simulink model "RBCM_Model"  (R2024b)
settings: Solver=FixedStepAuto  StartTime=0.0  StopTime=10.0  RelTol=1e-3
PreLoadFcn:
  | % NXP_MBDT_S32K3 callback: DO NOT REMOVE
  | mbd_s32k3.common.nxp.model_callbacks.preLoadFcn();
PostLoadFcn:
  | % NXP_MBDT_S32K3 callback: DO NOT REMOVE
  | mbd_s32k3.common.nxp.model_callbacks.postLoadFcn();
InitFcn:
  | % NXP_MBDT_S32K3 callback: DO NOT REMOVE
  | mbd_s32k3.common.nxp.model_callbacks.initFcn();
undefined symbols (not defined in the file or in its folder): AccuFanPwr_hHsd3ch2, BspdPwr_lHsd1ch2, BuzzerPwr_lHsd3ch3, DevicePwr_12v_lHsd1ch1, DevicePwr_hHsd1ch2, DrsPwr_8v_lHsd3ch1, hHsd_Diagnose_AdcBuffer, ILPwr_hHsd1ch1, lHsd_Diagnose_AdcBuffer, LoggerPwr_lHsd1ch3, PumpFan1_hHsd4ch1, PumpFan2_hHsd4ch2, PumpPwr_hHsd3ch1, RGBLED0state, TaillightPwr_lHsd3ch4, TempSensorPwr_lHsd1ch4
libraries: mbd_s32k3_io_library x127, simulink x48, canmsglib x8, mbd_s32k3_communication_library x7, mbd_s32k3_isr_library x6, mbd_s32k3_cdd_library x3, mbd_s32k3_utility_library x1
(part 10 of 10)

== matlab function RBCM_Model/HSD诊断分析子系统/错误码转存单元2 ==
  data: index input uint8; u input uint8; y1 output uint8; y2 output uint8; y3 output uint8; y4 output uint8
function [y1, y2, y3, y4] = fcn2(index, u)

% 函数内部声明 可持续类型变量
persistent Y1 Y2 Y3 Y4
% 首先要判断persistent声明的变量是否是空
if isempty(Y1)
    Y1=uint8(0);
    Y2=uint8(0);
    Y3=uint8(0);
    Y4=uint8(0);
end

if index==0
    y1=u;
    y2=Y2;
    y3=Y3;
    y4=Y4;
elseif index==1
    y1=Y1;
    y2=u;
    y3=Y3;
    y4=Y4;
elseif index==2
    y1=Y1;
    y2=Y2;
    y3=u;
    y4=Y4;
elseif index==3
    y1=Y1;
    y2=Y2;
    y3=Y3;
    y4=u;
else
    y1=Y1;
    y2=Y2;
    y3=Y3;
    y4=Y4;
end

Y1=y1;
Y2=y2;
Y3=y3;
Y4=y4;

end

== stateflow chart RBCM_Model/控制状态机/Chart1 ==
  state A
  state A1
  (default) -> A
  A -> A1
  A1 -> A
  data: A output boolean [0..1]

== matlab function RBCM_Model/HSD诊断分析子系统/错误码转存单元3 ==
  data: index input uint8; u input uint8; y1 output uint8; y2 output uint8; y3 output uint8; y4 output uint8
function [y1, y2, y3, y4] = fcn2(index, u)

% 函数内部声明 可持续类型变量
persistent Y1 Y2 Y3 Y4
% 首先要判断persistent声明的变量是否是空
if isempty(Y1)
    Y1=uint8(0);
    Y2=uint8(0);
    Y3=uint8(0);
    Y4=uint8(0);
end

if index==0
    y1=u;
    y2=Y2;
    y3=Y3;
    y4=Y4;
elseif index==1
    y1=Y1;
    y2=u;
    y3=Y3;
    y4=Y4;
elseif index==2
    y1=Y1;
    y2=Y2;
    y3=u;
    y4=Y4;
elseif index==3
    y1=Y1;
    y2=Y2;
    y3=Y3;
    y4=u;
else
    y1=Y1;
    y2=Y2;
    y3=Y3;
    y4=Y4;
end

Y1=y1;
Y2=y2;
Y3=y3;
Y4=y4;

end

== matlab function RBCM_Model/HSD诊断分析子系统/触发器5 ==
  data: y output uint8; counter input uint8; u2 input uint8
  events: fcncall output FUNCTION_CALL_EVENT
function y = fcn(counter,u2)

% 函数内部声明 可持续类型变量 output
persistent i
persistent output  
% 首先要判断persistent声明的变量是否是空
if isempty(i)
    i  = 0;
end
if isempty(output)
    output  = 0;
end

% 自递增
i=i+1;
output=output+1;

%分频计数值溢出
if i>=counter
    %输出值溢出
    if output>=u2
        output=0;
    end

    %输出值
    y = uint8(output);

    %生成触发，触发ADC采集
    fcncall;

    i=0;
else
    y=uint8(output);    %不生成触发
end

end

== matlab function RBCM_Model/HSD诊断分析子系统/诊断数据转存单元5 ==
  data: index input uint8; u input uint16; y1 output uint16; y2 output uint16; y3 output uint16; y4 output uint16
function [y1, y2, y3, y4] = fcn2(index, u)

% 函数内部声明 可持续类型变量
persistent Y1 Y2 Y3 Y4
% 首先要判断persistent声明的变量是否是空
if isempty(Y1)
    Y1=uint16(0);
    Y2=uint16(0);
    Y3=uint16(0);
    Y4=uint16(0);
end

if index==0
    y1=u;
    y2=Y2;
    y3=Y3;
    y4=Y4;
elseif index==1
    y1=Y1;
    y2=u;
    y3=Y3;
    y4=Y4;
elseif index==2
    y1=Y1;
    y2=Y2;
    y3=u;
    y4=Y4;
elseif index==3
    y1=Y1;
    y2=Y2;
    y3=Y3;
    y4=u;
else
    y1=Y1;
    y2=Y2;
    y3=Y3;
    y4=Y4;
end

Y1=y1;
Y2=y2;
Y3=y3;
Y4=y4;

end

== matlab function RBCM_Model/HSD诊断分析子系统/错误码转存单元4 ==
  data: index input uint8; u input uint8; y1 output uint8; y2 output uint8; y3 output uint8; y4 output uint8
function [y1, y2, y3, y4] = fcn2(index, u)

% 函数内部声明 可持续类型变量
persistent Y1 Y2 Y3 Y4
% 首先要判断persistent声明的变量是否是空
if isempty(Y1)
    Y1=uint8(0);
    Y2=uint8(0);
    Y3=uint8(0);
    Y4=uint8(0);
end

if index==0
    y1=u;
    y2=Y2;
    y3=Y3;
    y4=Y4;
elseif index==1
    y1=Y1;
    y2=u;
    y3=Y3;
    y4=Y4;
elseif index==2
    y1=Y1;
    y2=Y2;
    y3=u;
    y4=Y4;
elseif index==3
    y1=Y1;
    y2=Y2;
    y3=Y3;
    y4=u;
else
    y1=Y1;
    y2=Y2;
    y3=Y3;
    y4=Y4;
end

Y1=y1;
Y2=y2;
Y3=y3;
Y4=y4;

end

== matlab function RBCM_Model/HSD诊断分析子系统/数据转存单元2 ==
  data: index input uint8; u input uint8; y1 output uint8; y2 output uint8
function [y1, y2] = fcn2(index, u)

% 函数内部声明 可持续类型变量
persistent Y1 Y2
% 首先要判断persistent声明的变量是否是空
if isempty(Y1)
    Y1=uint8(0);
    Y2=uint8(0);
end

if index==0
    y1=u;
    y2=Y2;
elseif index==1
    y1=Y1;
    y2=u;
else
    y1=Y1;
    y2=Y2;
end

Y1=y1;
Y2=y2;

end

== matlab function RBCM_Model/HSD诊断分析子系统/数据转存单元3 ==
  data: index input uint8; u input uint16; y1 output uint16; y2 output uint16
function [y1, y2] = fcn2(index, u)

% 函数内部声明 可持续类型变量
persistent Y1 Y2
% 首先要判断persistent声明的变量是否是空
if isempty(Y1)
    Y1=uint16(0);
    Y2=uint16(0);
end

if index==0
    y1=u;
    y2=Y2;
elseif index==1
    y1=Y1;
    y2=u;
else
    y1=Y1;
    y2=Y2;
end

Y1=y1;
Y2=y2;

end

== matlab function RBCM_Model/HSD诊断分析子系统/触发器6 ==
  data: y output uint8; counter input uint8; u2 input uint8
  events: fcncall output FUNCTION_CALL_EVENT
function y = fcn(counter,u2)

% 函数内部声明 可持续类型变量 output
persistent i
persistent output  
% 首先要判断persistent声明的变量是否是空
if isempty(i)
    i  = 0;
end
if isempty(output)
    output  = 0;
end

% 自递增
i=i+1;
output=output+1;

%分频计数值溢出
if i>=counter
    %输出值溢出
    if output>=u2
        output=0;
    end

    %输出值
    y = uint8(output);

    %生成触发，触发ADC采集
    fcncall;

    i=0;
else
    y=uint8(output);    %不生成触发
end

end

== matlab function RBCM_Model/HSD诊断分析子系统/数据转存单元4 ==
  data: index input uint8; u input uint8; y1 output uint8; y2 output uint8
function [y1, y2] = fcn2(index, u)

% 函数内部声明 可持续类型变量
persistent Y1 Y2
% 首先要判断persistent声明的变量是否是空
if isempty(Y1)
    Y1=uint8(0);
    Y2=uint8(0);
end

if index==0
    y1=u;
    y2=Y2;
elseif index==1
    y1=Y1;
    y2=u;
else
    y1=Y1;
    y2=Y2;
end

Y1=y1;
Y2=y2;

end

== stateflow chart RBCM_Model/指令报文解码器/Chart1 ==
  state A
  state A1
  (default) -> A
  A -> A1
  A1 -> A
  data: A output boolean [0..1]

== matlab function RBCM_Model/HSD诊断分析子系统/数据转存单元5 ==
  data: index input uint8; u input uint16; y1 output uint16; y2 output uint16
function [y1, y2] = fcn2(index, u)

% 函数内部声明 可持续类型变量
persistent Y1 Y2
% 首先要判断persistent声明的变量是否是空
if isempty(Y1)
    Y1=uint16(0);
    Y2=uint16(0);
end

if index==0
    y1=u;
    y2=Y2;
elseif index==1
    y1=Y1;
    y2=u;
else
    y1=Y1;
    y2=Y2;
end

Y1=y1;
Y2=y2;

end

== matlab function RBCM_Model/HSD诊断分析子系统/数据转存单元6 ==
  data: index input uint8; u input uint8; y1 output uint8; y2 output uint8
function [y1, y2] = fcn2(index, u)

% 函数内部声明 可持续类型变量
persistent Y1 Y2
% 首先要判断persistent声明的变量是否是空
if isempty(Y1)
    Y1=uint8(0);
    Y2=uint8(0);
end

if index==0
    y1=u;
    y2=Y2;
elseif index==1
    y1=Y1;
    y2=u;
else
    y1=Y1;
    y2=Y2;
end

Y1=y1;
Y2=y2;

end

== matlab function RBCM_Model/HSD诊断分析子系统/数据转存单元7 ==
  data: index input uint8; u input uint16; y1 output uint16; y2 output uint16
function [y1, y2] = fcn2(index, u)

% 函数内部声明 可持续类型变量
persistent Y1 Y2
% 首先要判断persistent声明的变量是否是空
if isempty(Y1)
    Y1=uint16(0);
    Y2=uint16(0);
end

if index==0
    y1=u;
    y2=Y2;
elseif index==1
    y1=Y1;
    y2=u;
else
    y1=Y1;
    y2=Y2;
end

Y1=y1;
Y2=y2;

end

== matlab function RBCM_Model/HSD诊断分析子系统/触发器7 ==
  data: y output uint8; counter input uint8; u2 input uint8
  events: fcncall output FUNCTION_CALL_EVENT
function y = fcn(counter,u2)

% 函数内部声明 可持续类型变量 output
persistent i
persistent output  
% 首先要判断persistent声明的变量是否是空
if isempty(i)
    i  = 0;
end
if isempty(output)
    output  = 0;
end

% 自递增
i=i+1;
output=output+1;

%分频计数值溢出
if i>=counter
    %输出值溢出
    if output>=u2
        output=0;
    end

    %输出值
    y = uint8(output);

    %生成触发，触发ADC采集
    fcncall;

    i=0;
else
    y=uint8(output);    %不生成触发
end

end

== matlab function RBCM_Model/HSD诊断分析子系统/触发器8 ==
  data: y output uint8; counter input uint8; u2 input uint8
  events: fcncall output FUNCTION_CALL_EVENT
function y = fcn(counter,u2)

% 函数内部声明 可持续类型变量 output
persistent i
persistent output  
% 首先要判断persistent声明的变量是否是空
if isempty(i)
    i  = 0;
end
if isempty(output)
    output  = 0;
end

% 自递增
i=i+1;
output=output+1;

%分频计数值溢出
if i>=counter
    %输出值溢出
    if output>=u2
        output=0;
    end

    %输出值
    y = uint8(output);

    %生成触发，触发ADC采集
    fcncall;

    i=0;
else
    y=uint8(output);    %不生成触发
end

end

== matlab function RBCM_Model/HSD诊断分析子系统/数据转存单元8 ==
  data: index input uint8; u input uint8; y1 output uint8; y2 output uint8
function [y1, y2] = fcn2(index, u)

% 函数内部声明 可持续类型变量
persistent Y1 Y2
% 首先要判断persistent声明的变量是否是空
if isempty(Y1)
    Y1=uint8(0);
    Y2=uint8(0);
end

if index==0
    y1=u;
    y2=Y2;
elseif index==1
    y1=Y1;
    y2=u;
else
    y1=Y1;
    y2=Y2;
end

Y1=y1;
Y2=y2;

end

== matlab function RBCM_Model/HSD诊断分析子系统/数据转存单元9 ==
  data: index input uint8; u input uint16; y1 output uint16; y2 output uint16
function [y1, y2] = fcn2(index, u)

% 函数内部声明 可持续类型变量
persistent Y1 Y2
% 首先要判断persistent声明的变量是否是空
if isempty(Y1)
    Y1=uint16(0);
    Y2=uint16(0);
end

if index==0
    y1=u;
    y2=Y2;
elseif index==1
    y1=Y1;
    y2=u;
else
    y1=Y1;
    y2=Y2;
end

Y1=y1;
Y2=y2;

end

== matlab function RBCM_Model/HSD诊断分析子系统/触发器9 ==
  data: y output uint8; counter input uint8; u2 input uint8
  events: fcncall output FUNCTION_CALL_EVENT
function y = fcn(counter,u2)

% 函数内部声明 可持续类型变量 output
persistent i
persistent output  
% 首先要判断persistent声明的变量是否是空
if isempty(i)
    i  = 0;
end
if isempty(output)
    output  = 0;
end

% 自递增
i=i+1;
output=output+1;

%分频计数值溢出
if i>=counter
    %输出值溢出
    if output>=u2
        output=0;
    end

    %输出值
    y = uint8(output);

    %生成触发，触发ADC采集
    fcncall;

    i=0;
else
    y=uint8(output);    %不生成触发
end

end

== matlab function RBCM_Model/HSD诊断分析子系统/数据转存单元10 ==
  data: index input uint8; u input uint8; y1 output uint8; y2 output uint8
function [y1, y2] = fcn2(index, u)

% 函数内部声明 可持续类型变量
persistent Y1 Y2
% 首先要判断persistent声明的变量是否是空
if isempty(Y1)
    Y1=uint8(0);
    Y2=uint8(0);
end

if index==0
    y1=u;
    y2=Y2;
elseif index==1
    y1=Y1;
    y2=u;
else
    y1=Y1;
    y2=Y2;
end

Y1=y1;
Y2=y2;

end

== stateflow chart RBCM_Model/HSD驱动子系统/Subsystem1/Chart19 ==
  settings: description=寄存上一次的操作状态，同则不再操作，异才操作
  state High
    en:register=1
    du:register=1
  state Low
    en:register=0
    du:register=0
  (default) -> High
  High -> Low : [[bit==0]&[bit~=bit0]]{bit0=bit}
  Low -> High : [[bit==1]&[bit~=bit0]]{bit0=bit}
  data: bit input; register output

== matlab function RBCM_Model/HSD诊断分析子系统/数据转存单元12 ==
  data: index input uint8; u input uint16; y1 output uint16; y2 output uint16
function [y1, y2] = fcn2(index, u)

% 函数内部声明 可持续类型变量
persistent Y1 Y2
% 首先要判断persistent声明的变量是否是空
if isempty(Y1)
    Y1=uint16(0);
    Y2=uint16(0);
end

if index==0
    y1=u;
    y2=Y2;
elseif index==1
    y1=Y1;
    y2=u;
else
    y1=Y1;
    y2=Y2;
end

Y1=y1;
Y2=y2;

end

== matlab function RBCM_Model/HSD诊断分析子系统/触发器10 ==
  data: y output uint8; counter input uint8; u2 input uint8
  events: fcncall output FUNCTION_CALL_EVENT
function y = fcn(counter,u2)

% 函数内部声明 可持续类型变量 output
persistent i
persistent output  
% 首先要判断persistent声明的变量是否是空
if isempty(i)
    i  = 0;
end
if isempty(output)
    output  = 0;
end

% 自递增
i=i+1;
output=output+1;

%分频计数值溢出
if i>=counter
    %输出值溢出
    if output>=u2
        output=0;
    end

    %输出值
    y = uint8(output);

    %生成触发，触发ADC采集
    fcncall;

    i=0;
else
    y=uint8(output);    %不生成触发
end

end

== stateflow chart RBCM_Model/4G通信控制状态机1 ==
  settings: executeAtInitialization=1
  state init
    counter=0;
  state first
    if signal==0
    output=A
    counter = counter + 1
    end
  state second
    if signal==0
    output=B
    counter = counter + 1
    end
  state third
    if signal==0
    output=C
    counter = counter + 1
    end
  state fourth
    if signal==0
    output=D
    counter = counter + 1
    end
  state msgsend
  (default) -> init
  init -> first : timer_event[enable==1]{output=A}
  first -> init [order 2] : [enable==0||counter>=5]
  first -> second [order 1] : timer_event[signal==2]{output=B,counter=0}
  msgsend -> init [order 1] : [enable==0||counter>=5]
  fourth -> init [order 2] : [enable==0||counter>=5]
  second -> init [order 1] : [enable==0||counter>=5]
  second -> third [order 2] : timer_event[signal==2]{output=C,counter=0}
  third -> fourth : timer_event[signal==2]{output=D,counter=0}
  fourth -> msgsend [order 1] : timer_event[signal==2]{output=stringin,counter=0}
  msgsend -> msgsend [order 2] : timer_event{output=stringin}
  data: signal input uint32; enable input uint8; B local string ='AT+QMTOPEN=0,"2ac4d9928b.st1.iotda-device.cn-east-3.myhuaweicloud.com",1883'; C local string ='AT+QMTCONN=0,"E10_10101010_0_0_2024112708","E10_10101010","70cb096b1e95f2f5f6fa4a703d88b56f5d4bc5062f406b1091639f697a62929d"'; D local string ='AT+QMTSUB=0,1,"wute/car/test",2'; output output string; stringin input string; counter local uint8 size=1; A local string ="AT"
  events: timer_event input FUNCTION_CALL_EVENT

== matlab function RBCM_Model/Subsystem13/Subsystem/HsdDriveCommand Struct1 ==
  data: HsdDriveCommands output Bus: Bus_Hsd_Drive_Commands
function HsdDriveCommands = fcn

HsdDriveCommands.DevicePwr_12v_lHsd1ch1 = uint8(1);
HsdDriveCommands.BspdPwr_lHsd1ch2 = uint8(1);
HsdDriveCommands.LoggerPwr_lHsd1ch3 = uint8(1);
HsdDriveCommands.TempSensorPwr_lHsd1ch4 = uint8(1);

HsdDriveCommands.DevicePwr_12v_lHsd2ch1 = uint8(1);
HsdDriveCommands.VcuPwr_lHsd2ch2 = uint8(1);
HsdDriveCommands.Fireon_Pwr_lHsd2ch3 = uint8(1);
HsdDriveCommands.DsbdPwr_lHsd2ch4 = uint8(1);

HsdDriveCommands.DrsPwr_8v_lHsd3ch1 = uint8(1);
HsdDriveCommands.DevicePwr_lHsd3ch2 = uint8(1);
HsdDriveCommands.BuzzerPwr_lHsd3ch3 = uint8(1);
HsdDriveCommands.TaillightPwr_lHsd3ch4 = uint8(1);

HsdDriveCommands.DevicePwr_5v_lHsd4ch1 = uint8(1);
HsdDriveCommands.AccuUbr_lHsd4ch2 = uint8(1);
HsdDriveCommands.AccuPwr_lHsd4ch3 = uint8(1);
HsdDriveCommands.BduPwr_lHsd4ch4 = uint8(1);

HsdDriveCommands.DevicePwr_5v_lHsd5ch1 = uint8(1);
HsdDriveCommands.McuUbr_lHsd5ch2 = uint8(1);
HsdDriveCommands.EnergeMeterPwr_lHsd5ch3 = uint8(1);
HsdDriveCommands.TsalrPwr_lHsd5ch4 = uint8(1);


HsdDriveCommands.ILPwr_hHsd1ch1 = uint8(1);
HsdDriveCommands.DevicePwr_hHsd1ch2 = uint8(1);

HsdDriveCommands.VcuUbr_hHsd2ch1 = uint8(1);
HsdDriveCommands.Device_hHsd2ch2 = uint8(1);

HsdDriveCommands.PumpPwr_hHsd3ch1 = uint8(1);
HsdDriveCommands.AccuFanPwr_hHsd3ch2 = uint8(1);

HsdDriveCommands.PumpFan1_hHsd4ch1 = uint8(1);
HsdDriveCommands.PumpFan2_hHsd4ch2 = uint8(1);

HsdDriveCommands.DevicePwr_hHsd5ch1 = uint8(1);
HsdDriveCommands.DevicePwr_hHsd5ch2 = uint8(1);

HsdDriveCommands.DevicePwr_hHsd6ch1 = uint8(1);
HsdDriveCommands.DevicePwr_hHsd6ch2 = uint8(1);

== matlab function RBCM_Model/Subsystem9/Add '\r\n' ==
  data: u input; y output
function y = fcn(u)

y = [u 10 13];

== stateflow chart RBCM_Model/控制状态机/4G通信控制状态机 ==
  settings: executeAtInitialization=1
  state init
  state first
    if signal==0
    output=B
    end
  state second
    if signal==0
    output=C
    end
  state third
    if signal==0
    output=D
    end
  state end
    endflag=0
  (default) -> init
  init -> first : [signal==2&&enable==1]{output=B}
  first -> init [order 2] : [timer>=5||enable==0]
  first -> second [order 1] : [signal==2]{output=C}
  end -> init : [timer>=5||enable==0]
  third -> init [order 2] : [timer>=5||enable==0]
  second -> init [order 2] : [timer>=5||enable==0]
  second -> third [order 1] : [signal==2]{output=D}
  third -> end [order 1] : [signal==2]
  data: signal input uint32; enable input uint8; timer input uint8; B local string ='AT+QMTOPEN=0,"2ac4d9928b.st1.iotda-device.cn-east-3.myhuaweicloud.com",1883'; C local string ='AT+QMTCONN=0,"E10_10101010_0_0_2024112708","E10_10101010","70cb096b1e95f2f5f6fa4a703d88b56f5d4bc5062f406b1091639f697a62929d"'; D local string ='AT+QMTSUB=0,1,"wute/car/test",2'; output output string; endflag output uint8 [0..1] =1; stringin input string
  events: rx_event input FUNCTION_CALL_EVENT; timer_event input FUNCTION_CALL_EVENT
